simulink model "mdl"  (R2019b)
settings: Solver=VariableStepAuto  StartTime=0.0  StopTime=200  RelTol=1e-3
undefined symbols (not defined in the file): ABS, g, Jw, K, mv, rw, situation, T, v0
settings Model: Creator=bnier  LastModifiedBy=bnier

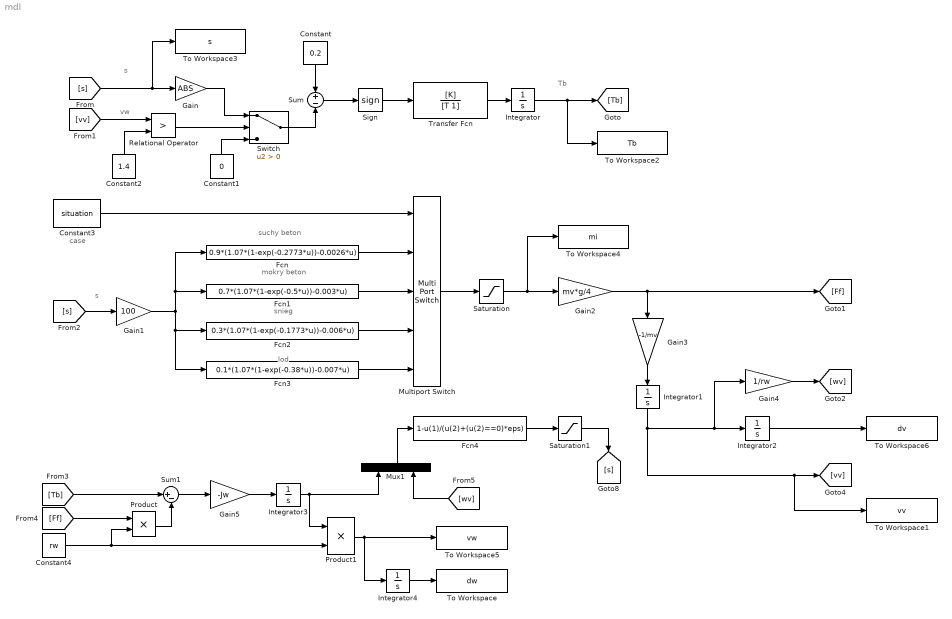
== system mdl ==
  note: s
  note: vw
  note: s
  note: Tb
  note: case
  note: snieg
  note: lod
  note: mokry beton
  note: suchy beton
  Constant : Constant  Value=0.2
  Constant1 : Constant  Value=0
  Constant2 : Constant  Value=1.4
  Constant3 : Constant  Value=situation
  Constant4 : Constant  Value=rw
  Fcn : Fcn  Expr=0.9*(1.07*(1-exp(-0.2773*u))-0.0026*u)
  Fcn1 : Fcn  Expr=0.7*(1.07*(1-exp(-0.5*u))-0.003*u)
  Fcn2 : Fcn  Expr=0.3*(1.07*(1-exp(-0.1773*u))-0.006*u)
  Fcn3 : Fcn  Expr=0.1*(1.07*(1-exp(-0.38*u))-0.007*u)
  Fcn4 : Fcn  Expr=1-u(1)/(u(2)+(u(2)==0)*eps)
  Gain : Gain  Gain=ABS
  Gain1 : Gain  Gain=100
  Gain2 : Gain  Gain=mv*g/4
  Gain3 : Gain  Gain=-1/mv
  Gain4 : Gain  Gain=1/rw
  Gain5 : Gain  Gain=-Jw
  Integrator : Integrator  LimitOutput=on  UpperSaturationLimit=2000  LowerSaturationLimit=0
  Integrator1 : Integrator  InitialCondition=v0  LimitOutput=on  UpperSaturationLimit=1000  LowerSaturationLimit=0.001
  Integrator2 : Integrator
  Integrator3 : Integrator  InitialCondition=v0/rw  LimitOutput=on  UpperSaturationLimit=1000  LowerSaturationLimit=0
  Integrator4 : Integrator
  Multiport Switch : MultiPortSwitch  Inputs=4
  Mux1 : Mux  Inputs=2
  Product : Product
  Product1 : Product
  Relational Operator : RelationalOperator  Operator=>  OutDataTypeStr=boolean  RndMeth=Simplest
  Saturation : Saturate  UpperLimit=1  LowerLimit=0
  Saturation1 : Saturate  UpperLimit=1  LowerLimit=0
  Sign : Signum
  Sum : Sum  Inputs=+|-
  Sum1 : Sum  Inputs=|+-
  Switch : Switch  Criteria=u2 > Threshold
  To Workspace : ToWorkspace  VariableName=dw  SaveFormat=Timeseries  SampleTime=-1
  To Workspace1 : ToWorkspace  VariableName=vv  SaveFormat=Timeseries  SampleTime=-1
  To Workspace2 : ToWorkspace  VariableName=Tb  SaveFormat=Timeseries  SampleTime=-1
  To Workspace3 : ToWorkspace  VariableName=s  SaveFormat=Timeseries  SampleTime=-1
  To Workspace4 : ToWorkspace  VariableName=mi  SaveFormat=Timeseries  SampleTime=-1
  To Workspace5 : ToWorkspace  VariableName=vw  SaveFormat=Timeseries  SampleTime=-1
  To Workspace6 : ToWorkspace  VariableName=dv  SaveFormat=Timeseries  SampleTime=-1
  Transfer Fcn : TransferFcn  Numerator=[K]  Denominator=[T 1]
  wires:
  Sign/1 -> Transfer Fcn/1
  [s] -> To Workspace3/1, Gain/1
  Integrator/1 -> [Tb], To Workspace2/1
  Gain/1 -> Switch/1
  Constant2/1 -> Relational Operator/2
  Transfer Fcn/1 -> Integrator/1
  Sum/1 -> Sign/1
  Constant1/1 -> Switch/3
  Switch/1 -> Sum/2
  Relational Operator/1 -> Switch/2
  [vv] -> Relational Operator/1
  Constant/1 -> Sum/1
  Fcn3/1 -> Multiport Switch/5
  Fcn/1 -> Multiport Switch/2
  Fcn2/1 -> Multiport Switch/4
  Gain1/1 -> Fcn3/1, Fcn2/1, Fcn1/1, Fcn/1
  Fcn1/1 -> Multiport Switch/3
  Multiport Switch/1 -> Saturation/1
  Constant3/1 -> Multiport Switch/1
  [s] -> Gain1/1
  Integrator1/1 -> [vv], To Workspace1/1, Gain4/1, Integrator2/1
  Gain4/1 -> [wv]
  Gain3/1 -> Integrator1/1
  Gain2/1 -> [Ff], Gain3/1
  Saturation/1 -> Gain2/1, To Workspace4/1
  Integrator2/1 -> To Workspace6/1
  Product1/1 -> Integrator4/1, To Workspace5/1
  Integrator4/1 -> To Workspace/1
  Integrator3/1 -> Mux1/1, Product1/1
  Sum1/1 -> Gain5/1
  [Ff] -> Product/1
  Constant4/1 -> Product1/2, Product/2
  Gain5/1 -> Integrator3/1
  Product/1 -> Sum1/2
  [Tb] -> Sum1/1
  Mux1/1 -> Fcn4/1
  Saturation1/1 -> [s]
  Fcn4/1 -> Saturation1/1
  [wv] -> Mux1/2
